simulink model "PMSM_SMC2"  (R2022b)
settings: Solver=ode23tb  StartTime=0.0  StopTime=1  FixedStep=Ts  RelTol=1e-4  EnableMultiTasking=on
InitFcn:
  | Ts = 10e-6;
  | 
  | R = 2.875;
  | Ld = 8.2e-3;
  | Lq = 8.2e-3;
  | Pn = 4;
  | flux = 0.175;
  | alpha1=15;
  | alpha2=9;
  | e=0.0005;
  | B = 0;
  | J = 0.003;
  | a=-(B/J);
  | b=(3*Pn*flux)/(2*J);
  | kq1=100;
  | kq2=80;
undefined symbols (not defined in the file): DiscIntNeverNeededParam, k1, k2
libraries: slpidlib x2, simulink x2, spsPermanentMagnetSynchronousMachineLib x1, powerlib_extras x1, spsUniversalBridgeLib x1, spsDCVoltageSourceLib x1, sps_lib x1
(part 1 of 2)
settings Model: Creator=SUN  LastModifiedBy=hl
settings SolverCC: ZeroCrossControl=DisableAll  AlgebraicLoopSolver=TrustRegion
settings DataIOCC: LimitDataPoints=on  SaveFormat=Array  SignalLoggingSaveFormat=ModelDataLogs  ReturnWorkspaceOutputs=off
settings OptimizationCC: ExpressionDepthLimit=2147483647  InitFltsAndDblsToZero=on  LifeSpan=inf
settings DebuggingCC: UnderspecifiedInitializationDetection=Classic  MergeDetectMultiDrivingBlocksExec=none  SolverPrmCheckMsg=warning  FcnCallInpInsideContextMsg=warning  UnconnectedInputMsg=warning  UnconnectedOutputMsg=warning  UnconnectedLineMsg=warning  StateNameClashWarn=warning  SFUnexpectedBacktrackingDiag=warning  SFNoUnconditionalDefaultTransitionDiag=warning  SFMachineParentedDataDiag=warning  ArithmeticOperatorsInVariantConditions=warning
settings HardwareCC: ProdBitPerPointer=32  ProdBitPerSizeT=32  ProdBitPerPtrDiffT=32  ProdLargestAtomicFloat=None  ProdIntDivRoundTo=Undefined  ProdEndianess=Unspecified  ProdWordSize=32  ProdHWDeviceType=32-bit Generic
settings ModelReferenceCC: EnableRefExpFcnMdlSchedulingChecks=on  PropagateSignalLabelsOutOfModel=off
settings SFSimCC: SimUseLocalCustomCode=off  CustomCodeUndefinedFunction=UseInterfaceOnly
settings RTWCC: RTWUseLocalCustomCode=off
settings CodeAppCC: StateflowObjectComments=on
settings GRTTargetCC: TargetLangStandard=C89/C90 (ANSI)  CombineOutputUpdateFcns=off  GRTInterface=on
settings ConfigComp: CovMetricSettings=dw  CovSaveCumulativeToWorkspaceVar=on  CovSaveSingleToWorkspaceVar=on  CovExternalEMLEnable=off  CovSFcnEnable=off
settings SimscapeCC: SimscapeNormalizeSystem=off

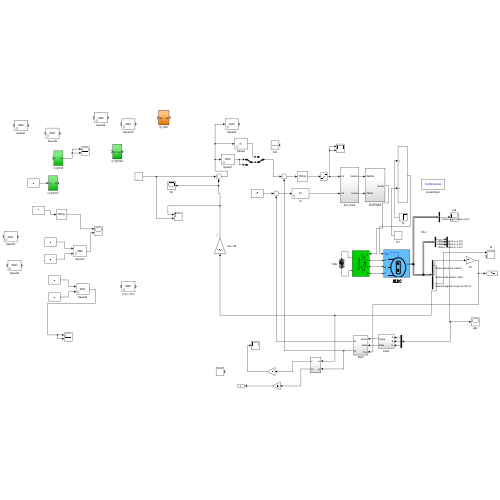
[thumbnail: Simulink's stored preview of the top-level diagram]
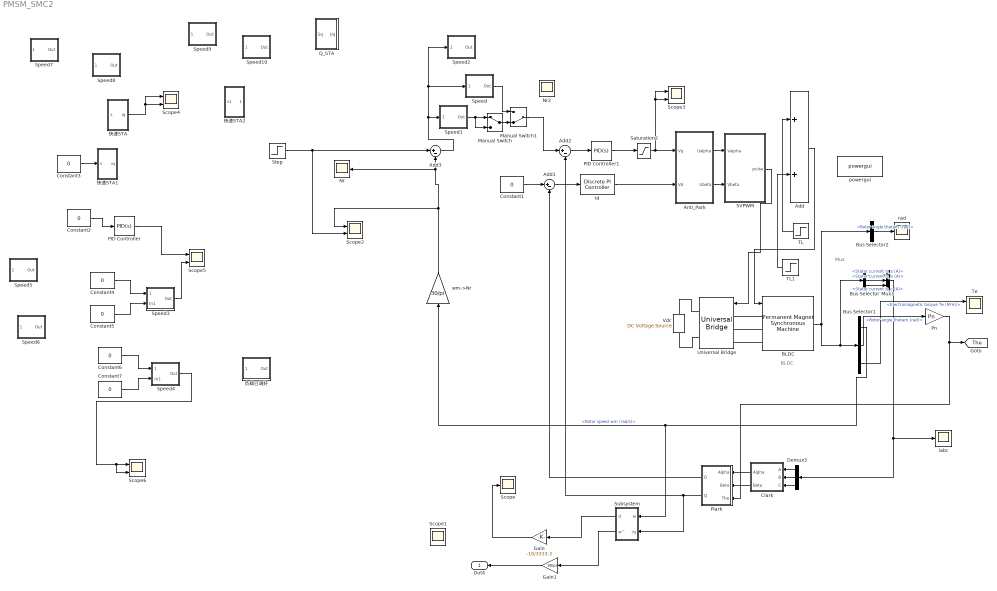
== system PMSM_SMC2 ==
  note: BLDC
  note: Mux
  Add : Sum
  Add1 : Sum  Inputs=|+-
  Add2 : Sum  Inputs=|+-
  Add3 : Sum  Inputs=|+-
  Anti_Park : Subsystem
  BLDC : spsPermanentMagnetSynchronousMachineLib/Permanent Magnet Synchronous Machine  NbPhases=3  FluxDistribution=Sinusoidal  RotorType=Salient-pole  MechanicalLoad=Torque Tm  PresetModel=No  ShowDetailedParameters=on  MeasurementBus=off  Resistance=2.875  Inductance=8.5e-3  dqInductances=[8.5e-3,8.5e-3]  La=0.000835  MachineConstant=Flux linkage established by magnets (V.s)  Flux=0.175  VoltageCst=126.966  TorqueCst=1.05  Flat=120  Mechanical=[0.003 0.008 4 0]  PolePairs=3  InitialConditions=[0,0, 0,0]  InitialConditions5ph=[0 0 0 0 0 0]  RefAngle=Aligned with phase A axis (original Park)  IterativeDiscreteModel=Trapezoidal non iterative  TsBlock=-1  TsPowergui=0
  Bus Selector : BusSelector  OutputSignals=Stator current is_a (A),Stator current is_b (A),Stator current is_c (A)
  Bus Selector1 : BusSelector  OutputSignals=Rotor speed wm (rad/s),Rotor angle thetam (rad),Electromagnetic torque Te (N*m)
  Bus Selector2 : BusSelector  OutputSignals=Rotor angle thetam (rad)
  Clark : Subsystem
  Constant{1..7} (7 alike) : Constant  Value=0
  Demux3 : Demux  Outputs=3
  Gain : Gain  Gain=-10/3333.3
  Gain1 : Gain  Gain=30/pi
  Id : powerlib_extras/Discrete  Control Blocks/Discrete PI Controller  Kp=Ld*2000  Ki=R*2000  Par_Limits=[311*0.9*sqrt(1/3) -311*0.9*sqrt(1/3)]  Init=0  Ts=Ts
  Manual Switch : ManualSwitch
  Manual Switch1 : ManualSwitch  CurrentSetting=0
  Mux3 : Mux  Inputs=3
  Nr : Scope
  Nr2 : Scope
  PID Controller : slpidlib/PID Controller  Controller=PID  Form=Parallel  TimeDomain=Continuous-time  UseExternalTs=off  SampleTime=-1  IntegratorMethod=Forward Euler  FilterMethod=Forward Euler  ControllerParametersSource=internal  P=60  I=10  UseKiTs=off  D=0  N=100  UseFilter=on  TunerSelectOption=Transfer Function Based (PID Tuner App)  InitialConditionSource=internal  InitialConditionForIntegrator=0  InitialConditionForFilter=0  DifferentiatorICPrevScaledInput=0  ExternalReset=none  TrackingMode=off  Kt=1  LimitOutput=off  SatLimitsSource=internal  UpperSaturationLimit=inf  LowerSaturationLimit=-inf  LinearizeAsGain=on  AntiWindupMode=none  Kb=1  LimitIntegrator=off  UpperIntegratorSaturationLimit=inf  LowerIntegratorSaturationLimit=-inf  POutMin=[]  POutMax=[]  IOutMin=[]  IOutMax=[]  DOutMin=[]  DOutMax=[]  NOutMin=[]  NOutMax=[]  SumOutMin=[]  SumOutMax=[]  SaturationOutMin=[]  SaturationOutMax=[]  PParamMin=[]  PParamMax=[]  IParamMin=[]  IParamMax=[]  DParamMin=[]  DParamMax=[]  NParamMin=[]  NParamMax=[]  KbParamMin=[]  KbParamMax=[]  KtParamMin=[]  KtParamMax=[]  KbOutMin=[]  KbOutMax=[]  KtOutMin=[]  KtOutMax=[]  IntegratorOutMin=[]  IntegratorOutMax=[]  FilterOutMin=[]  FilterOutMax=[]  SumI1OutMin=[]  SumI1OutMax=[]  SumI2OutMin=[]  SumI2OutMax=[]  SumI3OutMin=[]  SumI3OutMax=[]  SumI4OutMin=[]  SumI4OutMax=[]  SumDOutMin=[]  SumDOutMax=[]  DifferentiatorOutMin=[]  DifferentiatorOutMax=[]  FilterDiffOutCoefMin=[]  FilterDiffOutCoefMax=[]  ReciprocalOutMin=[]  ReciprocalOutMax=[]  SumDenOutMin=[]  SumDenOutMax=[]  SumNumOutMin=[]  SumNumOutMax=[]  DivideOutMin=[]  DivideOutMax=[]  UdiffTsProdOutMin=[]  UdiffTsProdOutMax=[]  NTsProdOutMin=[]  NTsProdOutMax=[]  UintegralTsProdOutMin=[]  UintegralTsProdOutMax=[]  UngainTsProdOutMin=[]  UngainTsProdOutMax=[]  ClampingZeroOutDataTypeStr=Inherit: Inherit via back propagation  ClampingZeroOutMin=[]  ClampingZeroOutMax=[]  FilterDenConstantOutDataTypeStr=Inherit: Inherit via back propagation  FilterDenConstantOutMin=[]  FilterDenConstantOutMax=[]  PCopyOutDataTypeStr=Inherit: Inherit via back propagation  PCopyOutMin=[]  PCopyOutMax=[]  NCopyOutDataTypeStr=Inherit: Inherit via back propagation  NCopyOutMin=[]  NCopyOutMax=[]  IntegratorContinuousStateAttributes=''  IntegratorStateMustResolveToSignalObject=off  IntegratorRTWStateStorageClass=Auto  FilterContinuousStateAttributes=''  FilterStateMustResolveToSignalObject=off  FilterRTWStateStorageClass=Auto  ParallelPVariant=InternalParameters  IdealPVariant=Disabled  IVariant=InternalParameters  DVariant=InternalParameters  IntegratorVariant=Continuous  SatVariant=Disabled  AWVariant=Passthrough  PCopyVariant=Disabled  TRVariant=Disabled  FdbkBlocksVariant=Forward  IdealPFdbkVariant=Disabled  SatFdbkVariant=Disabled  DerivativeFilterVariant=ContFilter  NVariant=InternalParameters  NCopyVariant=Disabled  FilterICVariant=InternalICsFilter  IntegratorICVariant=InternalICs  ExternalResetVariant=Disabled  TRSumVariant=Passthrough  SumFdbkVariant=Disabled  SumVariant=Sum_PID  TsampFilterVariant=InternalTs  TsampNgainVariant=Passthrough  TsampIntegralVariant=Passthrough  ExternalSaturationOutDataTypeStr=Inherit: Same as second input
  PID Controller1 : slpidlib/PID Controller  Controller=PID  Form=Parallel  TimeDomain=Continuous-time  UseExternalTs=off  SampleTime=-1  IntegratorMethod=Forward Euler  FilterMethod=Forward Euler  ControllerParametersSource=internal  P=60  I=10  UseKiTs=off  D=0  N=100  UseFilter=on  TunerSelectOption=Transfer Function Based (PID Tuner App)  InitialConditionSource=internal  InitialConditionForIntegrator=0  InitialConditionForFilter=0  DifferentiatorICPrevScaledInput=0  ExternalReset=none  TrackingMode=off  Kt=1  LimitOutput=off  SatLimitsSource=internal  UpperSaturationLimit=inf  LowerSaturationLimit=-inf  LinearizeAsGain=on  AntiWindupMode=none  Kb=1  LimitIntegrator=off  UpperIntegratorSaturationLimit=inf  LowerIntegratorSaturationLimit=-inf  POutMin=[]  POutMax=[]  IOutMin=[]  IOutMax=[]  DOutMin=[]  DOutMax=[]  NOutMin=[]  NOutMax=[]  SumOutMin=[]  SumOutMax=[]  SaturationOutMin=[]  SaturationOutMax=[]  PParamMin=[]  PParamMax=[]  IParamMin=[]  IParamMax=[]  DParamMin=[]  DParamMax=[]  NParamMin=[]  NParamMax=[]  KbParamMin=[]  KbParamMax=[]  KtParamMin=[]  KtParamMax=[]  KbOutMin=[]  KbOutMax=[]  KtOutMin=[]  KtOutMax=[]  IntegratorOutMin=[]  IntegratorOutMax=[]  FilterOutMin=[]  FilterOutMax=[]  SumI1OutMin=[]  SumI1OutMax=[]  SumI2OutMin=[]  SumI2OutMax=[]  SumI3OutMin=[]  SumI3OutMax=[]  SumI4OutMin=[]  SumI4OutMax=[]  SumDOutMin=[]  SumDOutMax=[]  DifferentiatorOutMin=[]  DifferentiatorOutMax=[]  FilterDiffOutCoefMin=[]  FilterDiffOutCoefMax=[]  ReciprocalOutMin=[]  ReciprocalOutMax=[]  SumDenOutMin=[]  SumDenOutMax=[]  SumNumOutMin=[]  SumNumOutMax=[]  DivideOutMin=[]  DivideOutMax=[]  UdiffTsProdOutMin=[]  UdiffTsProdOutMax=[]  NTsProdOutMin=[]  NTsProdOutMax=[]  UintegralTsProdOutMin=[]  UintegralTsProdOutMax=[]  UngainTsProdOutMin=[]  UngainTsProdOutMax=[]  ClampingZeroOutDataTypeStr=Inherit: Inherit via back propagation  ClampingZeroOutMin=[]  ClampingZeroOutMax=[]  FilterDenConstantOutDataTypeStr=Inherit: Inherit via back propagation  FilterDenConstantOutMin=[]  FilterDenConstantOutMax=[]  PCopyOutDataTypeStr=Inherit: Inherit via back propagation  PCopyOutMin=[]  PCopyOutMax=[]  NCopyOutDataTypeStr=Inherit: Inherit via back propagation  NCopyOutMin=[]  NCopyOutMax=[]  IntegratorContinuousStateAttributes=''  IntegratorStateMustResolveToSignalObject=off  IntegratorRTWStateStorageClass=Auto  FilterContinuousStateAttributes=''  FilterStateMustResolveToSignalObject=off  FilterRTWStateStorageClass=Auto  ParallelPVariant=InternalParameters  IdealPVariant=Disabled  IVariant=InternalParameters  DVariant=InternalParameters  IntegratorVariant=Continuous  SatVariant=Disabled  AWVariant=Passthrough  PCopyVariant=Disabled  TRVariant=Disabled  FdbkBlocksVariant=Forward  IdealPFdbkVariant=Disabled  SatFdbkVariant=Disabled  DerivativeFilterVariant=ContFilter  NVariant=InternalParameters  NCopyVariant=Disabled  FilterICVariant=InternalICsFilter  IntegratorICVariant=InternalICs  ExternalResetVariant=Disabled  TRSumVariant=Passthrough  SumFdbkVariant=Disabled  SumVariant=Sum_PID  TsampFilterVariant=InternalTs  TsampNgainVariant=Passthrough  TsampIntegralVariant=Passthrough  ExternalSaturationOutDataTypeStr=Inherit: Same as second input
  Plark : Subsystem
  Pn : Gain  Gain=Pn
  Q_STA : Subsystem
  SVPWM : Subsystem
  Saturation2 : Saturate  UpperLimit=380  LowerLimit=-400  SampleTime=Ts
  Scope : Scope
  Scope1 : Scope
  Scope{2..6} (5 alike) : Scope  NumInputPorts=2
  Speed : Subsystem  AncestorBlock=|  DialogController=POWERSYS.PowerSysDialog  mask(Discrete PI Controller){Kpw=0.14, Kiw=0.14*50, Ba=0.013, Par_Limits=[30 -30], Init=0, Ts=Ts}
      | powerlib_extras/Discrete 
      | Control Blocks/Discrete
      | PI Controller
      mask prompts: Kpw "Proportional gain (Kp):"; Kiw "Integral gain (Ki):"; Ba "feedback gain (Ba)"; Par_Limits "Output limits: [ Upper   Lower ]"; Init "Output initial value:"; Ts "Sample time:"
      mask help: This block implements a discrete PI controller.
      mask init:
      | UpperLimit=Par_Limits(1);
      | LowerLimit=Par_Limits(2);
      | power_initmask();
      settings: LibrarySourceBlock=|
      | powerlib_extras/Discrete
      | Control Blocks/Discrete
      | PI Controller
      mask Help: This block is part of a subset of blocks in the Extras library that does not have documentation associated with it, other than the block mask description.
      mask Display: disp('PI');
  Speed1 : Subsystem  AncestorBlock=|  DialogController=POWERSYS.PowerSysDialog  mask(Discrete PI Controller){C=294.3, Mu=200, q=500, Par_Limits=[30 -30], Init=0, Ts=Ts}
      | powerlib_extras/Discrete 
      | Control Blocks/Discrete
      | PI Controller
      mask prompts: C "Gain (c):"; Mu "Gain (Mu):"; q "Gain (q)"; Par_Limits "Output limits: [ Upper   Lower ]"; Init "Output initial value:"; Ts "Sample time:"
      mask help: This block implements a discrete PI controller.
      mask init:
      | UpperLimit=Par_Limits(1);
      | LowerLimit=Par_Limits(2);
      | power_initmask();
      settings: LibrarySourceBlock=|
      | powerlib_extras/Discrete
      | Control Blocks/Discrete
      | PI Controller
      mask Help: This block is part of a subset of blocks in the Extras library that does not have documentation associated with it, other than the block mask description.
      mask Display: disp('SMC');
  Speed10 : Subsystem  AncestorBlock=|  DialogController=POWERSYS.PowerSysDialog  mask(Discrete PI Controller){C=294.3, Mu=200, q=500, Par_Limits=[30 -30], Init=0, Ts=Ts}
      | powerlib_extras/Discrete 
      | Control Blocks/Discrete
      | PI Controller
      mask prompts: C "Gain (c):"; Mu "Gain (Mu):"; q "Gain (q)"; Par_Limits "Output limits: [ Upper   Lower ]"; Init "Output initial value:"; Ts "Sample time:"
      mask help: This block implements a discrete PI controller.
      mask init:
      | UpperLimit=Par_Limits(1);
      | LowerLimit=Par_Limits(2);
      | power_initmask();
      settings: LibrarySourceBlock=|
      | powerlib_extras/Discrete
      | Control Blocks/Discrete
      | PI Controller
      mask Help: This block is part of a subset of blocks in the Extras library that does not have documentation associated with it, other than the block mask description.
      mask Display: disp('SMC');
  Speed2 : Subsystem  AncestorBlock=|  DialogController=POWERSYS.PowerSysDialog  mask(Discrete PI Controller){C=50, Mu=500, q=1000, Par_Limits=[30 -30], Init=0, Ts=Ts}
      | powerlib_extras/Discrete 
      | Control Blocks/Discrete
      | PI Controller
      mask prompts: C "Gain (c):"; Mu "Gain (Mu):"; q "Gain (q)"; Par_Limits "Output limits: [ Upper   Lower ]"; Init "Output initial value:"; Ts "Sample time:"
      mask help: This block implements a discrete PI controller.
      mask init:
      | UpperLimit=Par_Limits(1);
      | LowerLimit=Par_Limits(2);
      | power_initmask();
      settings: LibrarySourceBlock=|
      | powerlib_extras/Discrete
      | Control Blocks/Discrete
      | PI Controller
      mask Help: This block is part of a subset of blocks in the Extras library that does not have documentation associated with it, other than the block mask description.
      mask Display: disp('SMC');
  Speed3 : Subsystem  AncestorBlock=|  DialogController=POWERSYS.PowerSysDialog  mask(Discrete PI Controller){C=605, Mu=200, q=410, Par_Limits=[30 -30], Init=0, Ts=Ts}
      | powerlib_extras/Discrete 
      | Control Blocks/Discrete
      | PI Controller
      mask prompts: C "Gain (c):"; Mu "Gain (Mu):"; q "Gain (q)"; Par_Limits "Output limits: [ Upper   Lower ]"; Init "Output initial value:"; Ts "Sample time:"
      mask help: This block implements a discrete PI controller.
      mask init:
      | UpperLimit=Par_Limits(1);
      | LowerLimit=Par_Limits(2);
      | power_initmask();
      settings: LibrarySourceBlock=|
      | powerlib_extras/Discrete
      | Control Blocks/Discrete
      | PI Controller
      mask Help: This block is part of a subset of blocks in the Extras library that does not have documentation associated with it, other than the block mask description.
      mask Display: disp('SMC');
  Speed4 : Subsystem  AncestorBlock=|  DialogController=POWERSYS.PowerSysDialog  mask(Discrete PI Controller){C=600, Mu=200, q=403.81, Par_Limits=[30 -30], Init=0, Ts=Ts}
      | powerlib_extras/Discrete 
      | Control Blocks/Discrete
      | PI Controller
      mask prompts: C "Gain (c):"; Mu "Gain (Mu):"; q "Gain (q)"; Par_Limits "Output limits: [ Upper   Lower ]"; Init "Output initial value:"; Ts "Sample time:"
      mask help: This block implements a discrete PI controller.
      mask init:
      | UpperLimit=Par_Limits(1);
      | LowerLimit=Par_Limits(2);
      | power_initmask();
      settings: LibrarySourceBlock=|
      | powerlib_extras/Discrete
      | Control Blocks/Discrete
      | PI Controller
      mask Help: This block is part of a subset of blocks in the Extras library that does not have documentation associated with it, other than the block mask description.
      mask Display: disp('SMC');
  Speed5 : Subsystem  AncestorBlock=|  DialogController=POWERSYS.PowerSysDialog  mask(Discrete PI Controller){C=370, Mu=200, q=500, Par_Limits=[30 -30], Init=0, Ts=Ts}
      | powerlib_extras/Discrete 
      | Control Blocks/Discrete
      | PI Controller
      mask prompts: C "Gain (c):"; Mu "Gain (Mu):"; q "Gain (q)"; Par_Limits "Output limits: [ Upper   Lower ]"; Init "Output initial value:"; Ts "Sample time:"
      mask help: This block implements a discrete PI controller.
      mask init:
      | UpperLimit=Par_Limits(1);
      | LowerLimit=Par_Limits(2);
      | power_initmask();
      settings: LibrarySourceBlock=|
      | powerlib_extras/Discrete
      | Control Blocks/Discrete
      | PI Controller
      mask Help: This block is part of a subset of blocks in the Extras library that does not have documentation associated with it, other than the block mask description.
      mask Display: disp('SMC');
  Speed6 : Subsystem  AncestorBlock=|  DialogController=POWERSYS.PowerSysDialog  mask(Discrete PI Controller){C=500, Mu=200, q=300, Par_Limits=[30 -30], Init=0, Ts=Ts}
      | powerlib_extras/Discrete 
      | Control Blocks/Discrete
      | PI Controller
      mask prompts: C "Gain (c):"; Mu "Gain (Mu):"; q "Gain (q)"; Par_Limits "Output limits: [ Upper   Lower ]"; Init "Output initial value:"; Ts "Sample time:"
      mask help: This block implements a discrete PI controller.
      mask init:
      | UpperLimit=Par_Limits(1);
      | LowerLimit=Par_Limits(2);
      | power_initmask();
      settings: LibrarySourceBlock=|
      | powerlib_extras/Discrete
      | Control Blocks/Discrete
      | PI Controller
      mask Help: This block is part of a subset of blocks in the Extras library that does not have documentation associated with it, other than the block mask description.
      mask Display: disp('SMC');
  Speed7 : Subsystem  AncestorBlock=|  DialogController=POWERSYS.PowerSysDialog  mask(Discrete PI Controller){C=195, Mu=200, q=400, Par_Limits=[30 -30], Init=0, Ts=Ts}
      | powerlib_extras/Discrete 
      | Control Blocks/Discrete
      | PI Controller
      mask prompts: C "Gain (c):"; Mu "Gain (Mu):"; q "Gain (q)"; Par_Limits "Output limits: [ Upper   Lower ]"; Init "Output initial value:"; Ts "Sample time:"
      mask help: This block implements a discrete PI controller.
      mask init:
      | UpperLimit=Par_Limits(1);
      | LowerLimit=Par_Limits(2);
      | power_initmask();
      settings: LibrarySourceBlock=|
      | powerlib_extras/Discrete
      | Control Blocks/Discrete
      | PI Controller
      mask Help: This block is part of a subset of blocks in the Extras library that does not have documentation associated with it, other than the block mask description.
      mask Display: disp('SMC');
  Speed8 : Subsystem  AncestorBlock=|  DialogController=POWERSYS.PowerSysDialog  mask(Discrete PI Controller){C=195, Mu=200, q=300, Par_Limits=[30 -30], Init=0, Ts=Ts}
      | powerlib_extras/Discrete 
      | Control Blocks/Discrete
      | PI Controller
      mask prompts: C "Gain (c):"; Mu "Gain (Mu):"; q "Gain (q)"; Par_Limits "Output limits: [ Upper   Lower ]"; Init "Output initial value:"; Ts "Sample time:"
      mask help: This block implements a discrete PI controller.
      mask init:
      | UpperLimit=Par_Limits(1);
      | LowerLimit=Par_Limits(2);
      | power_initmask();
      settings: LibrarySourceBlock=|
      | powerlib_extras/Discrete
      | Control Blocks/Discrete
      | PI Controller
      mask Help: This block is part of a subset of blocks in the Extras library that does not have documentation associated with it, other than the block mask description.
      mask Display: disp('SMC');
  Speed9 : Subsystem  AncestorBlock=|  DialogController=POWERSYS.PowerSysDialog  mask(Discrete PI Controller){C=150, Mu=200, q=200, Par_Limits=[30 -30], Init=0, Ts=Ts}
      | powerlib_extras/Discrete 
      | Control Blocks/Discrete
      | PI Controller
      mask prompts: C "Gain (c):"; Mu "Gain (Mu):"; q "Gain (q)"; Par_Limits "Output limits: [ Upper   Lower ]"; Init "Output initial value:"; Ts "Sample time:"
      mask help: This block implements a discrete PI controller.
      mask init:
      | UpperLimit=Par_Limits(1);
      | LowerLimit=Par_Limits(2);
      | power_initmask();
      settings: LibrarySourceBlock=|
      | powerlib_extras/Discrete
      | Control Blocks/Discrete
      | PI Controller
      mask Help: This block is part of a subset of blocks in the Extras library that does not have documentation associated with it, other than the block mask description.
      mask Display: disp('SMC');
  Step : Step  Time=0.6  Before=500  After=1000  SampleTime=0
  Subsystem : Subsystem
  TL : Step  Time=0.3  After=10  SampleTime=0
  TL1 : Step  Time=0.8  After=-5  SampleTime=0
  Te : Scope  NumInputPorts=2
  Universal Bridge : spsUniversalBridgeLib/Universal Bridge  Arms=3  SnubberResistance=1e5  SnubberCapacitance=inf  Device=IGBT / Diodes  Ron=1e-3  Lon=0  ForwardVoltages="[  0  0  ]"  ForwardVoltage=0  GTOparameters=[ 10e-6 , 20e-6 ]  IGBTparameters=[ 1e-6 , 2e-6 ]  Measurements=None  Measurements_2=None  converterType=Rectifier
  Vdc : spsDCVoltageSourceLib/DC Voltage Source  Amplitude=311  Measurements=None
  iabc : Scope
  powergui : sps_lib/powergui  SimulationMode=Continuous  SampleTime=Ts  frequency=60  Iterations=50  frequencyindice=0  Pbase=100e6  ErrMax=1e-4  UnitsV=kV  UnitsW=MW  buscounter=0  FunctionMessages=off  echomessages=off  EnableUseOfTLC=off  CurrentSourceSwitches=on  DisableSnubberDevices=off  DisableRonSwitches=off  DisableVfSwitches=off  DisplayEquations=off  AutomaticDiscreteSolvers=off  SolverType=Tustin/Backward Euler (TBE)  Interpol=off  ExternalGateDelay=off  methode=off  Ts=0  x0status=blocks  SPID=off  SwTol=0  HookPort=off  NonlinearTolerance=1e-4  nMaxIteration=100  ContinueOnMaxIteration=off  RestoreLinks=warning  ResistiveCurrentMeasurement=off  Frange=[0:2:500]  Ylog=off  Xlog=on  ShowGrid=off  save=off  variable=ZData  structure=0  ZoomFFT=on  StartTime=0.0  cycles=1  DisplayStyle=1  fundamental=60  FreqAxis=off  MaxFrequency=1000  frequencyindicesteady=1  RmsSteady=1  display=off
  rad : Scope
  wm->Nr : Gain  Gain=30/pi
  快速STA : Subsystem
  快速STA1 : Subsystem
  快速STA2 : Subsystem
  负载已调好 : Subsystem  AncestorBlock=|  DialogController=POWERSYS.PowerSysDialog  mask(Discrete PI Controller){C=515, Mu=200, q=450, Par_Limits=[30 -30], Init=0, Ts=Ts}
      | powerlib_extras/Discrete 
      | Control Blocks/Discrete
      | PI Controller
      mask prompts: C "Gain (c):"; Mu "Gain (Mu):"; q "Gain (q)"; Par_Limits "Output limits: [ Upper   Lower ]"; Init "Output initial value:"; Ts "Sample time:"
      mask help: This block implements a discrete PI controller.
      mask init:
      | UpperLimit=Par_Limits(1);
      | LowerLimit=Par_Limits(2);
      | power_initmask();
      settings: LibrarySourceBlock=|
      | powerlib_extras/Discrete
      | Control Blocks/Discrete
      | PI Controller
      mask Help: This block is part of a subset of blocks in the Extras library that does not have documentation associated with it, other than the block mask description.
      mask Display: disp('SMC');
  Out4 : Outport
  tag scope: The=global
  wires:
  Constant1/1 -> Add1/1
  wm->Nr/1 -> Add3/2, Nr/1, Scope2/1
  Id/1 -> Anti_Park/2(Vd)
  Pn/1 -> Plark/3(The), [The]
  SVPWM/1(pulse) -> Universal Bridge/1
  Mux3/1 -> Demux3/1, iabc/1
  Anti_Park/1(Ualpha) -> SVPWM/1(Valpha)
  Anti_Park/2(Ubeta) -> SVPWM/2(Vbeta)
  Bus Selector/1 -> Mux3/1  "<Stator current is_a (A)>"
  Bus Selector/3 -> Mux3/3  "<Stator current is_c (A)>"
  Bus Selector/2 -> Mux3/2  "<Stator current is_b (A)>"
  BLDC/1 -> Bus Selector/1, Bus Selector1/1, Bus Selector2/1
  Bus Selector1/3 -> Te/1  "<Electromagnetic torque Te (N*m)>"
  Bus Selector1/2 -> Pn/1  "<Rotor angle thetam (rad)>"
  Bus Selector1/1 -> Subsystem/1(w), wm->Nr/1  "<Rotor speed wm (rad/s)>"
  Bus Selector2/1 -> rad/1  "<Rotor angle thetam (rad)>"
  Add1/1 -> Id/1
  Saturation2/1 -> Anti_Park/1(Vq), Scope3/2, Scope3/1
  TL/1 -> Add/1
  TL1/1 -> Add/2
  Add/1 -> BLDC/1
  Constant2/1 -> PID Controller/1
  PID Controller/1 -> Scope5/1
  快速STA/1(iq) -> Scope4/1, Scope4/2
  Constant4/1 -> Speed3/1(Error)
  Constant5/1 -> Speed3/2(In1)
  Speed3/1(Out) -> Scope5/2
  Step/1 -> Scope2/2, Add3/1
  Constant6/1 -> Speed4/1(Error)
  Constant7/1 -> Speed4/2(In1)
  Speed4/1(Out) -> Scope6/2, Scope6/1
  Constant3/1 -> 快速STA1/1(s)
  Manual Switch/1 -> Manual Switch1/2
  Speed1/1(Out) -> Manual Switch/2, Manual Switch/1
  Demux3/2 -> Clark/2(B)
  Plark/2(Q) -> Add2/2, Subsystem/2(iq)
  Demux3/3 -> Clark/3(C)
  Clark/2(Beta) -> Plark/2(Beta)
  Subsystem/2(w^) -> Gain1/1
  Clark/1(Alpha) -> Plark/1(Alpha)
  Gain1/1 -> Out4/1
  Subsystem/1(d) -> Gain/1
  Demux3/1 -> Clark/1(A)
  Plark/1(D) -> Add1/2
  Gain/1 -> Scope/1
  Manual Switch1/1 -> Add2/1
  Add3/1 -> Speed/1(Error), Speed2/1(Error), Speed1/1(Error)
  Add2/1 -> PID Controller1/1
  PID Controller1/1 -> Saturation2/1
  Speed/1(Out) -> Manual Switch1/1
  connections:
  Universal Bridge/RConn1 -- Vdc/RConn1
  BLDC/LConn3 -- Universal Bridge/LConn3
  BLDC/LConn2 -- Universal Bridge/LConn2
  Universal Bridge/RConn2 -- Vdc/LConn1
  BLDC/LConn1 -- Universal Bridge/LConn1

== system PMSM_SMC2/Anti_Park ==
  Vq : Inport
  Vd : Inport  Port=2
  Fcn : Fcn  Expr=cos(u[1])*u[2]-sin(u[1])*u[3]
  Fcn1 : Fcn  Expr=sin(u[1])*u[2]+cos(u[1])*u[3]
  Mux1 : Mux  Inputs=3
  Ualpha : Outport  VectorParamsAs1DForOutWhenUnconnected=off
  Ubeta : Outport  Port=2  VectorParamsAs1DForOutWhenUnconnected=off
  wires:
  Fcn1/1 -> Ubeta/1
  Fcn/1 -> Ualpha/1
  Mux1/1 -> Fcn/1, Fcn1/1
  Vd/1 -> Mux1/2
  Vq/1 -> Mux1/3
  [The] -> Mux1/1

== system PMSM_SMC2/Clark ==
  A : Inport
  B : Inport  Port=2
  C : Inport  Port=3
  Mux : Mux  Inputs=3
  alpha : Fcn  Expr=(u(1)-0.5*(u(2)+u(3)))*2/3
  beta : Fcn  Expr=sqrt(3)/2*(u(2)-u(3))*2/3
  Alpha : Outport  VectorParamsAs1DForOutWhenUnconnected=off
  Beta : Outport  Port=2  VectorParamsAs1DForOutWhenUnconnected=off
  wires:
  alpha/1 -> Alpha/1
  B/1 -> Mux/2
  C/1 -> Mux/3
  A/1 -> Mux/1
  Mux/1 -> beta/1, alpha/1
  beta/1 -> Beta/1

== system PMSM_SMC2/Plark ==
  Alpha : Inport
  Beta : Inport  Port=2
  The : Inport  Port=3
  Mux : Mux  Inputs=3
  d : Fcn  Expr=u(1)*cos(u(3))+u(2)*sin(u(3))
  q : Fcn  Expr=-u(1)*sin(u(3))+u(2)*cos(u(3))
  D : Outport  VectorParamsAs1DForOutWhenUnconnected=off
  Q : Outport  Port=2  VectorParamsAs1DForOutWhenUnconnected=off
  wires:
  d/1 -> D/1
  Beta/1 -> Mux/2
  The/1 -> Mux/3
  Alpha/1 -> Mux/1
  Mux/1 -> q/1, d/1
  q/1 -> Q/1

== system PMSM_SMC2/Q_STA ==
  Sq : Inport
  Abs : Abs  SaturateOnIntegerOverflow=off
  Add : Sum
  Constant : Constant  Value=0.5
  Discrete-Time Integrator : DiscreteIntegrator  ICPrevOutput=DiscIntNeverNeededParam  ICPrevScaledInput=DiscIntNeverNeededParam
  Gain : Gain  Gain=100
  Gain1 : Gain  Gain=300
  Math Function : Math  Operator=pow  SignedPower=on
  Product : Product
  Sign : Signum
  Uq : Outport
  wires:
  Add/1 -> Uq/1
  Gain1/1 -> Discrete-Time Integrator/1
  Discrete-Time Integrator/1 -> Add/2
  Gain/1 -> Add/1
  Sq/1 -> Sign/1, Abs/1
  Product/1 -> Gain/1
  Sign/1 -> Gain1/1, Product/2
  Constant/1 -> Math Function/2
  Math Function/1 -> Product/1
  Abs/1 -> Math Function/1

== system PMSM_SMC2/SVPWM ==
  Valpha : Inport
  Vbeta : Inport  Port=2
  PWM : Subsystem
  Repeating Sequence : simulink/Sources/Repeating Sequence  rep_seq_t=[0 0.00005 0.0001]  rep_seq_y=[0 0.00005 0]
  Sector Caculate : Subsystem
  T1T1 Caculate : Subsystem
  Tcm Caculate : Subsystem
  Tpwm : Constant  Value=0.0001
  Vdc : Constant  Value=311
  XYZ Caculate : Subsystem
  pulse : Outport  VectorParamsAs1DForOutWhenUnconnected=off
  wires:
  PWM/1(PWM) -> pulse/1
  Repeating Sequence/1 -> PWM/1(In)
  Vbeta/1 -> XYZ Caculate/2(Ubeta), Sector Caculate/2(Ubeta)
  T1T1 Caculate/1(T1) -> Tcm Caculate/2(T1)
  Valpha/1 -> XYZ Caculate/1(Ualpha), Sector Caculate/1(Ualpha)
  T1T1 Caculate/2(T2) -> Tcm Caculate/3(T2)
  Sector Caculate/1("N ") -> Tcm Caculate/1(N), T1T1 Caculate/1(N)
  XYZ Caculate/1(XYZ) -> T1T1 Caculate/2(XYZ)
  Tpwm/1 -> XYZ Caculate/3(Ts), Tcm Caculate/4(Tpwm), T1T1 Caculate/3(Tpwm)
  Vdc/1 -> XYZ Caculate/4(Udc)
  Tcm Caculate/1(Tcm1 Tcm2 Tcm3) -> PWM/2(Tcm123)

== system PMSM_SMC2/Speed ==
  note: Discrete PID Controller
  note: Pierre Giroux, Gilbert Sybille
      | Power System Simulation Laboratory
      | IREQ, Hydro-Quebc
  Error : Inport  SampleTime=Ts
  Discrete-Time Integrator : DiscreteIntegrator  InitialCondition=Init  SampleTime=Ts  LimitOutput=on  UpperSaturationLimit=UpperLimit  LowerSaturationLimit=LowerLimit  ICPrevOutput=DiscIntNeverNeededParam  ICPrevScaledInput=DiscIntNeverNeededParam
  Kp1 : Gain  Gain=Ba  SaturateOnIntegerOverflow=on  SampleTime=Ts  OutDataTypeStr=Inherit: Same as input  ParamDataTypeStr=Inherit: Same as input
  Kp4 : Gain  Gain=Kpw  SaturateOnIntegerOverflow=on  SampleTime=Ts  OutDataTypeStr=Inherit: Same as input  ParamDataTypeStr=Inherit: Same as input
  Kp5 : Gain  Gain=Kiw  SaturateOnIntegerOverflow=on  SampleTime=Ts  OutDataTypeStr=Inherit: Same as input  ParamDataTypeStr=Inherit: Same as input
  Saturation2 : Saturate  UpperLimit=UpperLimit  LowerLimit=LowerLimit  SampleTime=Ts
  Sum6 : Sum  Inputs=++-  InputSameDT=on  SaturateOnIntegerOverflow=on  SampleTime=Ts  OutDataTypeStr=Inherit: Same as first input
  Zero-Order Hold : ZeroOrderHold  SampleTime=Ts
  Out : Outport  SampleTime=Ts  InitialOutput=0  VectorParamsAs1DForOutWhenUnconnected=off
  wires:
  Error/1 -> Kp1/1, Kp5/1, Kp4/1
  Zero-Order Hold/1 -> Sum6/1
  Saturation2/1 -> Out/1
  Discrete-Time Integrator/1 -> Sum6/2
  Kp4/1 -> Zero-Order Hold/1
  Kp5/1 -> Discrete-Time Integrator/1
  Sum6/1 -> Saturation2/1
  Kp1/1 -> Sum6/3

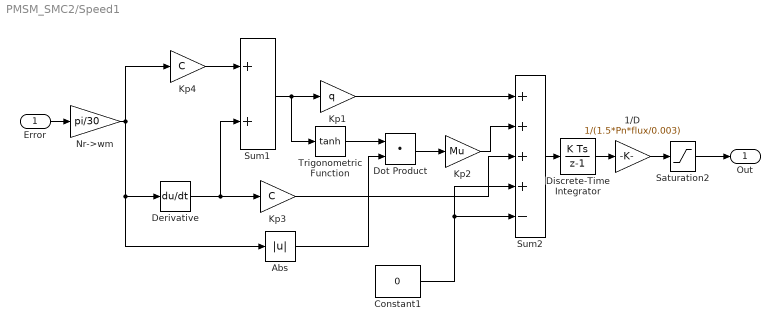
== system PMSM_SMC2/Speed1 ==
  Error : Inport  SampleTime=Ts
  1/D : Gain  Gain=1/(1.5*Pn*flux/0.003)  SaturateOnIntegerOverflow=on  SampleTime=Ts  OutDataTypeStr=Inherit: Same as input  ParamDataTypeStr=Inherit: Same as input
  Abs : Abs  SaturateOnIntegerOverflow=off
  Constant1 : Constant  Value=0
  Derivative : Derivative
  Discrete-Time Integrator : DiscreteIntegrator  InitialCondition=0.001  SampleTime=Ts  ICPrevOutput=DiscIntNeverNeededParam  ICPrevScaledInput=DiscIntNeverNeededParam
  Dot Product : DotProduct  OutDataTypeStr=Inherit: Inherit via internal rule
  Kp1 : Gain  Gain=q  SaturateOnIntegerOverflow=on  SampleTime=Ts  OutDataTypeStr=Inherit: Same as input  ParamDataTypeStr=Inherit: Same as input
  Kp2 : Gain  Gain=Mu  SaturateOnIntegerOverflow=on  SampleTime=Ts  OutDataTypeStr=Inherit: Same as input  ParamDataTypeStr=Inherit: Same as input
  Kp3 : Gain  Gain=C  SaturateOnIntegerOverflow=on  SampleTime=Ts  OutDataTypeStr=Inherit: Same as input  ParamDataTypeStr=Inherit: Same as input
  Kp4 : Gain  Gain=C  SaturateOnIntegerOverflow=on  SampleTime=Ts  OutDataTypeStr=Inherit: Same as input  ParamDataTypeStr=Inherit: Same as input
  Nr->wm : Gain  Gain=pi/30  SaturateOnIntegerOverflow=on  SampleTime=Ts  OutDataTypeStr=Inherit: Same as input  ParamDataTypeStr=Inherit: Same as input
  Saturation2 : Saturate  UpperLimit=UpperLimit  LowerLimit=LowerLimit  SampleTime=Ts
  Sum1 : Sum  InputSameDT=on  SaturateOnIntegerOverflow=on  SampleTime=Ts  OutDataTypeStr=Inherit: Same as first input
  Sum2 : Sum  Inputs=++++-  InputSameDT=on  SaturateOnIntegerOverflow=on  SampleTime=Ts  OutDataTypeStr=Inherit: Same as first input
  Trigonometric Function : Trigonometry  Operator=tanh
  Out : Outport  SampleTime=Ts  InitialOutput=0  VectorParamsAs1DForOutWhenUnconnected=off
  wires:
  Kp4/1 -> Sum1/1
  Saturation2/1 -> Out/1
  Error/1 -> Nr->wm/1
  Kp1/1 -> Sum2/1
  Sum1/1 -> Trigonometric Function/1, Kp1/1
  Kp2/1 -> Sum2/2
  Kp3/1 -> Sum2/3
  Nr->wm/1 -> Kp4/1, Abs/1, Derivative/1
  Derivative/1 -> Sum1/2, Kp3/1
  Sum2/1 -> Discrete-Time Integrator/1
  1/D/1 -> Saturation2/1
  Discrete-Time Integrator/1 -> 1/D/1
  Dot Product/1 -> Kp2/1
  Abs/1 -> Dot Product/2
  Trigonometric Function/1 -> Dot Product/1
  Constant1/1 -> Sum2/5, Sum2/4

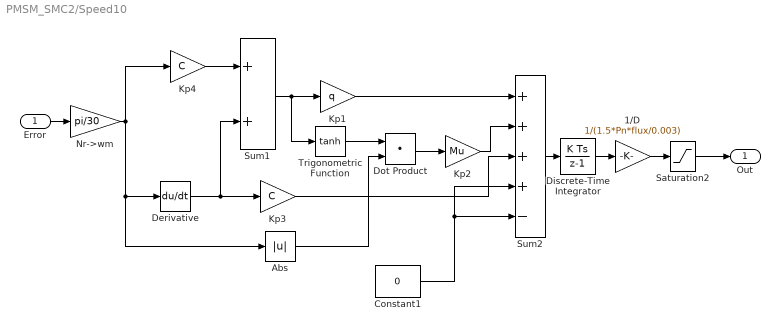
== system PMSM_SMC2/Speed10 ==
  Error : Inport  SampleTime=Ts
  1/D : Gain  Gain=1/(1.5*Pn*flux/0.003)  SaturateOnIntegerOverflow=on  SampleTime=Ts  OutDataTypeStr=Inherit: Same as input  ParamDataTypeStr=Inherit: Same as input
  Abs : Abs  SaturateOnIntegerOverflow=off
  Constant1 : Constant  Value=0
  Derivative : Derivative
  Discrete-Time Integrator : DiscreteIntegrator  InitialCondition=0.001  SampleTime=Ts  ICPrevOutput=DiscIntNeverNeededParam  ICPrevScaledInput=DiscIntNeverNeededParam
  Dot Product : DotProduct  OutDataTypeStr=Inherit: Inherit via internal rule
  Kp1 : Gain  Gain=q  SaturateOnIntegerOverflow=on  SampleTime=Ts  OutDataTypeStr=Inherit: Same as input  ParamDataTypeStr=Inherit: Same as input
  Kp2 : Gain  Gain=Mu  SaturateOnIntegerOverflow=on  SampleTime=Ts  OutDataTypeStr=Inherit: Same as input  ParamDataTypeStr=Inherit: Same as input
  Kp3 : Gain  Gain=C  SaturateOnIntegerOverflow=on  SampleTime=Ts  OutDataTypeStr=Inherit: Same as input  ParamDataTypeStr=Inherit: Same as input
  Kp4 : Gain  Gain=C  SaturateOnIntegerOverflow=on  SampleTime=Ts  OutDataTypeStr=Inherit: Same as input  ParamDataTypeStr=Inherit: Same as input
  Nr->wm : Gain  Gain=pi/30  SaturateOnIntegerOverflow=on  SampleTime=Ts  OutDataTypeStr=Inherit: Same as input  ParamDataTypeStr=Inherit: Same as input
  Saturation2 : Saturate  UpperLimit=UpperLimit  LowerLimit=LowerLimit  SampleTime=Ts
  Sum1 : Sum  InputSameDT=on  SaturateOnIntegerOverflow=on  SampleTime=Ts  OutDataTypeStr=Inherit: Same as first input
  Sum2 : Sum  Inputs=++++-  InputSameDT=on  SaturateOnIntegerOverflow=on  SampleTime=Ts  OutDataTypeStr=Inherit: Same as first input
  Trigonometric Function : Trigonometry  Operator=tanh
  Out : Outport  SampleTime=Ts  InitialOutput=0  VectorParamsAs1DForOutWhenUnconnected=off
  wires:
  Kp4/1 -> Sum1/1
  Saturation2/1 -> Out/1
  Error/1 -> Nr->wm/1
  Kp1/1 -> Sum2/1
  Sum1/1 -> Trigonometric Function/1, Kp1/1
  Kp2/1 -> Sum2/2
  Kp3/1 -> Sum2/3
  Nr->wm/1 -> Kp4/1, Abs/1, Derivative/1
  Derivative/1 -> Sum1/2, Kp3/1
  Sum2/1 -> Discrete-Time Integrator/1
  1/D/1 -> Saturation2/1
  Discrete-Time Integrator/1 -> 1/D/1
  Dot Product/1 -> Kp2/1
  Abs/1 -> Dot Product/2
  Trigonometric Function/1 -> Dot Product/1
  Constant1/1 -> Sum2/5, Sum2/4

== system PMSM_SMC2/Speed2 ==
  Error : Inport  SampleTime=Ts
  1/D : Gain  Gain=1/(1.5*Pn*flux/0.003)  SaturateOnIntegerOverflow=on  SampleTime=Ts  OutDataTypeStr=Inherit: Same as input  ParamDataTypeStr=Inherit: Same as input
  Discrete Derivative : simulink/Discrete/Discrete Derivative  gainval=1.0  ICPrevScaledInput=0.0  OutMin=[]  OutMax=[]  OutDataType=fixdt(1, 16)  OutScaling=2^-10  DoSatur=off
  Discrete-Time Integrator : DiscreteIntegrator  InitialCondition=0.001  SampleTime=Ts  ICPrevOutput=DiscIntNeverNeededParam  ICPrevScaledInput=DiscIntNeverNeededParam
  Kp1 : Gain  Gain=q  SaturateOnIntegerOverflow=on  SampleTime=Ts  OutDataTypeStr=Inherit: Same as input  ParamDataTypeStr=Inherit: Same as input
  Kp2 : Gain  Gain=Mu  SaturateOnIntegerOverflow=on  SampleTime=Ts  OutDataTypeStr=Inherit: Same as input  ParamDataTypeStr=Inherit: Same as input
  Kp3 : Gain  Gain=C  SaturateOnIntegerOverflow=on  SampleTime=Ts  OutDataTypeStr=Inherit: Same as input  ParamDataTypeStr=Inherit: Same as input
  Kp4 : Gain  Gain=C  SaturateOnIntegerOverflow=on  SampleTime=Ts  OutDataTypeStr=Inherit: Same as input  ParamDataTypeStr=Inherit: Same as input
  Nr->wm : Gain  Gain=pi/30  SaturateOnIntegerOverflow=on  SampleTime=Ts  OutDataTypeStr=Inherit: Same as input  ParamDataTypeStr=Inherit: Same as input
  Saturation2 : Saturate  UpperLimit=UpperLimit  LowerLimit=LowerLimit  SampleTime=Ts
  Sign : Signum
  Sum1 : Sum  InputSameDT=on  SaturateOnIntegerOverflow=on  SampleTime=Ts  OutDataTypeStr=Inherit: Same as first input
  Sum2 : Sum  Inputs=++-  InputSameDT=on  SaturateOnIntegerOverflow=on  SampleTime=Ts  OutDataTypeStr=Inherit: Same as first input
  Out : Outport  SampleTime=Ts  InitialOutput=0
  wires:
  Kp4/1 -> Sum1/1
  Saturation2/1 -> Out/1
  Discrete Derivative/1 -> Kp3/1, Sum1/2
  Sum2/1 -> Discrete-Time Integrator/1
  Error/1 -> Nr->wm/1
  Kp1/1 -> Sum2/1
  Sum1/1 -> Kp1/1, Sign/1
  Kp2/1 -> Sum2/2
  Kp3/1 -> Sum2/3
  1/D/1 -> Saturation2/1
  Discrete-Time Integrator/1 -> 1/D/1
  Nr->wm/1 -> Discrete Derivative/1, Kp4/1
  Sign/1 -> Kp2/1

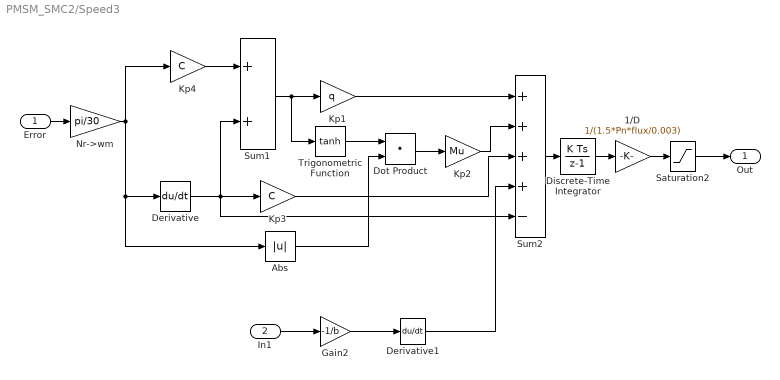
== system PMSM_SMC2/Speed3 ==
  Error : Inport  SampleTime=Ts
  In1 : Inport  Port=2
  1/D : Gain  Gain=1/(1.5*Pn*flux/0.003)  SaturateOnIntegerOverflow=on  SampleTime=Ts  OutDataTypeStr=Inherit: Same as input  ParamDataTypeStr=Inherit: Same as input
  Abs : Abs  SaturateOnIntegerOverflow=off
  Derivative : Derivative
  Derivative1 : Derivative
  Discrete-Time Integrator : DiscreteIntegrator  InitialCondition=0.001  SampleTime=Ts  ICPrevOutput=DiscIntNeverNeededParam  ICPrevScaledInput=DiscIntNeverNeededParam
  Dot Product : DotProduct  OutDataTypeStr=Inherit: Inherit via internal rule
  Gain2 : Gain  Gain=-1/b
  Kp1 : Gain  Gain=q  SaturateOnIntegerOverflow=on  SampleTime=Ts  OutDataTypeStr=Inherit: Same as input  ParamDataTypeStr=Inherit: Same as input
  Kp2 : Gain  Gain=Mu  SaturateOnIntegerOverflow=on  SampleTime=Ts  OutDataTypeStr=Inherit: Same as input  ParamDataTypeStr=Inherit: Same as input
  Kp3 : Gain  Gain=C  SaturateOnIntegerOverflow=on  SampleTime=Ts  OutDataTypeStr=Inherit: Same as input  ParamDataTypeStr=Inherit: Same as input
  Kp4 : Gain  Gain=C  SaturateOnIntegerOverflow=on  SampleTime=Ts  OutDataTypeStr=Inherit: Same as input  ParamDataTypeStr=Inherit: Same as input
  Nr->wm : Gain  Gain=pi/30  SaturateOnIntegerOverflow=on  SampleTime=Ts  OutDataTypeStr=Inherit: Same as input  ParamDataTypeStr=Inherit: Same as input
  Saturation2 : Saturate  UpperLimit=UpperLimit  LowerLimit=LowerLimit  SampleTime=Ts
  Sum1 : Sum  InputSameDT=on  SaturateOnIntegerOverflow=on  SampleTime=Ts  OutDataTypeStr=Inherit: Same as first input
  Sum2 : Sum  Inputs=++++-  InputSameDT=on  SaturateOnIntegerOverflow=on  SampleTime=Ts  OutDataTypeStr=Inherit: Same as first input
  Trigonometric Function : Trigonometry  Operator=tanh
  Out : Outport  SampleTime=Ts  InitialOutput=0  VectorParamsAs1DForOutWhenUnconnected=off
  wires:
  Kp4/1 -> Sum1/1
  Saturation2/1 -> Out/1
  Error/1 -> Nr->wm/1
  Kp1/1 -> Sum2/1
  Sum1/1 -> Trigonometric Function/1, Kp1/1
  Kp2/1 -> Sum2/2
  Kp3/1 -> Sum2/3
  Nr->wm/1 -> Kp4/1, Abs/1, Derivative/1
  Derivative/1 -> Sum2/5, Sum1/2, Kp3/1
  Sum2/1 -> Discrete-Time Integrator/1
  1/D/1 -> Saturation2/1
  Discrete-Time Integrator/1 -> 1/D/1
  Dot Product/1 -> Kp2/1
  Abs/1 -> Dot Product/2
  In1/1 -> Gain2/1
  Gain2/1 -> Derivative1/1
  Derivative1/1 -> Sum2/4
  Trigonometric Function/1 -> Dot Product/1

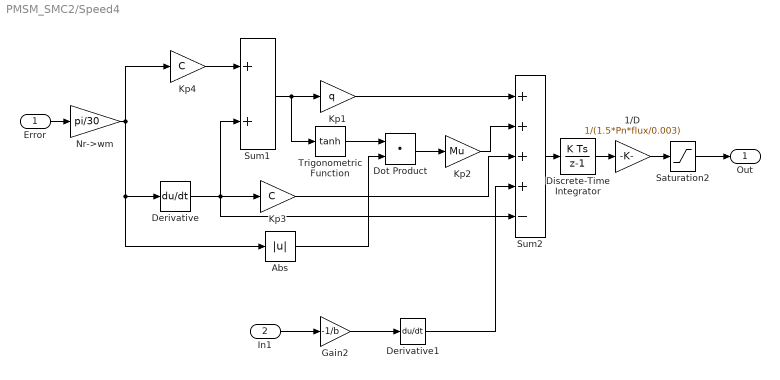
== system PMSM_SMC2/Speed4 ==
  Error : Inport  SampleTime=Ts
  In1 : Inport  Port=2
  1/D : Gain  Gain=1/(1.5*Pn*flux/0.003)  SaturateOnIntegerOverflow=on  SampleTime=Ts  OutDataTypeStr=Inherit: Same as input  ParamDataTypeStr=Inherit: Same as input
  Abs : Abs  SaturateOnIntegerOverflow=off
  Derivative : Derivative
  Derivative1 : Derivative
  Discrete-Time Integrator : DiscreteIntegrator  InitialCondition=0.001  SampleTime=Ts  ICPrevOutput=DiscIntNeverNeededParam  ICPrevScaledInput=DiscIntNeverNeededParam
  Dot Product : DotProduct  OutDataTypeStr=Inherit: Inherit via internal rule
  Gain2 : Gain  Gain=-1/b
  Kp1 : Gain  Gain=q  SaturateOnIntegerOverflow=on  SampleTime=Ts  OutDataTypeStr=Inherit: Same as input  ParamDataTypeStr=Inherit: Same as input
  Kp2 : Gain  Gain=Mu  SaturateOnIntegerOverflow=on  SampleTime=Ts  OutDataTypeStr=Inherit: Same as input  ParamDataTypeStr=Inherit: Same as input
  Kp3 : Gain  Gain=C  SaturateOnIntegerOverflow=on  SampleTime=Ts  OutDataTypeStr=Inherit: Same as input  ParamDataTypeStr=Inherit: Same as input
  Kp4 : Gain  Gain=C  SaturateOnIntegerOverflow=on  SampleTime=Ts  OutDataTypeStr=Inherit: Same as input  ParamDataTypeStr=Inherit: Same as input
  Nr->wm : Gain  Gain=pi/30  SaturateOnIntegerOverflow=on  SampleTime=Ts  OutDataTypeStr=Inherit: Same as input  ParamDataTypeStr=Inherit: Same as input
  Saturation2 : Saturate  UpperLimit=UpperLimit  LowerLimit=LowerLimit  SampleTime=Ts
  Sum1 : Sum  InputSameDT=on  SaturateOnIntegerOverflow=on  SampleTime=Ts  OutDataTypeStr=Inherit: Same as first input
  Sum2 : Sum  Inputs=++++-  InputSameDT=on  SaturateOnIntegerOverflow=on  SampleTime=Ts  OutDataTypeStr=Inherit: Same as first input
  Trigonometric Function : Trigonometry  Operator=tanh
  Out : Outport  SampleTime=Ts  InitialOutput=0  VectorParamsAs1DForOutWhenUnconnected=off
  wires:
  Kp4/1 -> Sum1/1
  Saturation2/1 -> Out/1
  Error/1 -> Nr->wm/1
  Kp1/1 -> Sum2/1
  Sum1/1 -> Trigonometric Function/1, Kp1/1
  Kp2/1 -> Sum2/2
  Kp3/1 -> Sum2/3
  Nr->wm/1 -> Kp4/1, Abs/1, Derivative/1
  Derivative/1 -> Sum2/5, Sum1/2, Kp3/1
  Sum2/1 -> Discrete-Time Integrator/1
  1/D/1 -> Saturation2/1
  Discrete-Time Integrator/1 -> 1/D/1
  Dot Product/1 -> Kp2/1
  Abs/1 -> Dot Product/2
  In1/1 -> Gain2/1
  Gain2/1 -> Derivative1/1
  Derivative1/1 -> Sum2/4
  Trigonometric Function/1 -> Dot Product/1

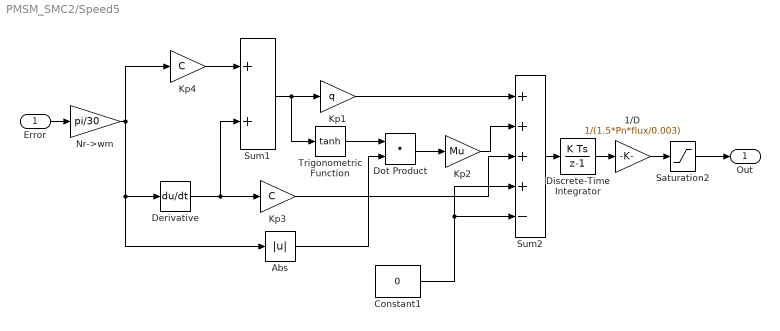
== system PMSM_SMC2/Speed5 ==
  Error : Inport  SampleTime=Ts
  1/D : Gain  Gain=1/(1.5*Pn*flux/0.003)  SaturateOnIntegerOverflow=on  SampleTime=Ts  OutDataTypeStr=Inherit: Same as input  ParamDataTypeStr=Inherit: Same as input
  Abs : Abs  SaturateOnIntegerOverflow=off
  Constant1 : Constant  Value=0
  Derivative : Derivative
  Discrete-Time Integrator : DiscreteIntegrator  InitialCondition=0.001  SampleTime=Ts  ICPrevOutput=DiscIntNeverNeededParam  ICPrevScaledInput=DiscIntNeverNeededParam
  Dot Product : DotProduct  OutDataTypeStr=Inherit: Inherit via internal rule
  Kp1 : Gain  Gain=q  SaturateOnIntegerOverflow=on  SampleTime=Ts  OutDataTypeStr=Inherit: Same as input  ParamDataTypeStr=Inherit: Same as input
  Kp2 : Gain  Gain=Mu  SaturateOnIntegerOverflow=on  SampleTime=Ts  OutDataTypeStr=Inherit: Same as input  ParamDataTypeStr=Inherit: Same as input
  Kp3 : Gain  Gain=C  SaturateOnIntegerOverflow=on  SampleTime=Ts  OutDataTypeStr=Inherit: Same as input  ParamDataTypeStr=Inherit: Same as input
  Kp4 : Gain  Gain=C  SaturateOnIntegerOverflow=on  SampleTime=Ts  OutDataTypeStr=Inherit: Same as input  ParamDataTypeStr=Inherit: Same as input
  Nr->wm : Gain  Gain=pi/30  SaturateOnIntegerOverflow=on  SampleTime=Ts  OutDataTypeStr=Inherit: Same as input  ParamDataTypeStr=Inherit: Same as input
  Saturation2 : Saturate  UpperLimit=UpperLimit  LowerLimit=LowerLimit  SampleTime=Ts
  Sum1 : Sum  InputSameDT=on  SaturateOnIntegerOverflow=on  SampleTime=Ts  OutDataTypeStr=Inherit: Same as first input
  Sum2 : Sum  Inputs=++++-  InputSameDT=on  SaturateOnIntegerOverflow=on  SampleTime=Ts  OutDataTypeStr=Inherit: Same as first input
  Trigonometric Function : Trigonometry  Operator=tanh
  Out : Outport  SampleTime=Ts  InitialOutput=0  VectorParamsAs1DForOutWhenUnconnected=off
  wires:
  Kp4/1 -> Sum1/1
  Saturation2/1 -> Out/1
  Error/1 -> Nr->wm/1
  Kp1/1 -> Sum2/1
  Sum1/1 -> Trigonometric Function/1, Kp1/1
  Kp2/1 -> Sum2/2
  Kp3/1 -> Sum2/3
  Nr->wm/1 -> Kp4/1, Abs/1, Derivative/1
  Derivative/1 -> Sum1/2, Kp3/1
  Sum2/1 -> Discrete-Time Integrator/1
  1/D/1 -> Saturation2/1
  Discrete-Time Integrator/1 -> 1/D/1
  Dot Product/1 -> Kp2/1
  Abs/1 -> Dot Product/2
  Trigonometric Function/1 -> Dot Product/1
  Constant1/1 -> Sum2/5, Sum2/4

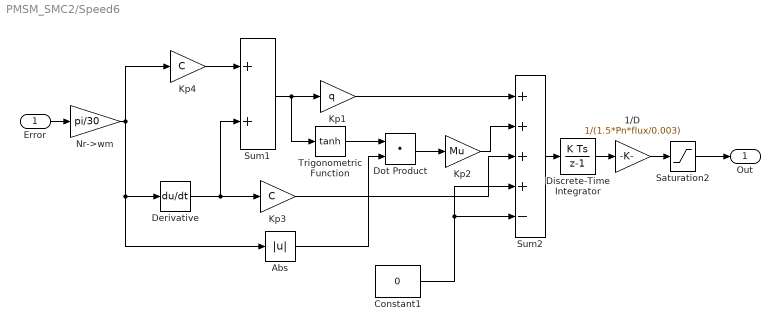
== system PMSM_SMC2/Speed6 ==
  Error : Inport  SampleTime=Ts
  1/D : Gain  Gain=1/(1.5*Pn*flux/0.003)  SaturateOnIntegerOverflow=on  SampleTime=Ts  OutDataTypeStr=Inherit: Same as input  ParamDataTypeStr=Inherit: Same as input
  Abs : Abs  SaturateOnIntegerOverflow=off
  Constant1 : Constant  Value=0
  Derivative : Derivative
  Discrete-Time Integrator : DiscreteIntegrator  InitialCondition=0.001  SampleTime=Ts  ICPrevOutput=DiscIntNeverNeededParam  ICPrevScaledInput=DiscIntNeverNeededParam
  Dot Product : DotProduct  OutDataTypeStr=Inherit: Inherit via internal rule
  Kp1 : Gain  Gain=q  SaturateOnIntegerOverflow=on  SampleTime=Ts  OutDataTypeStr=Inherit: Same as input  ParamDataTypeStr=Inherit: Same as input
  Kp2 : Gain  Gain=Mu  SaturateOnIntegerOverflow=on  SampleTime=Ts  OutDataTypeStr=Inherit: Same as input  ParamDataTypeStr=Inherit: Same as input
  Kp3 : Gain  Gain=C  SaturateOnIntegerOverflow=on  SampleTime=Ts  OutDataTypeStr=Inherit: Same as input  ParamDataTypeStr=Inherit: Same as input
  Kp4 : Gain  Gain=C  SaturateOnIntegerOverflow=on  SampleTime=Ts  OutDataTypeStr=Inherit: Same as input  ParamDataTypeStr=Inherit: Same as input
  Nr->wm : Gain  Gain=pi/30  SaturateOnIntegerOverflow=on  SampleTime=Ts  OutDataTypeStr=Inherit: Same as input  ParamDataTypeStr=Inherit: Same as input
  Saturation2 : Saturate  UpperLimit=UpperLimit  LowerLimit=LowerLimit  SampleTime=Ts
  Sum1 : Sum  InputSameDT=on  SaturateOnIntegerOverflow=on  SampleTime=Ts  OutDataTypeStr=Inherit: Same as first input
  Sum2 : Sum  Inputs=++++-  InputSameDT=on  SaturateOnIntegerOverflow=on  SampleTime=Ts  OutDataTypeStr=Inherit: Same as first input
  Trigonometric Function : Trigonometry  Operator=tanh
  Out : Outport  SampleTime=Ts  InitialOutput=0  VectorParamsAs1DForOutWhenUnconnected=off
  wires:
  Kp4/1 -> Sum1/1
  Saturation2/1 -> Out/1
  Error/1 -> Nr->wm/1
  Kp1/1 -> Sum2/1
  Sum1/1 -> Trigonometric Function/1, Kp1/1
  Kp2/1 -> Sum2/2
  Kp3/1 -> Sum2/3
  Nr->wm/1 -> Kp4/1, Abs/1, Derivative/1
  Derivative/1 -> Sum1/2, Kp3/1
  Sum2/1 -> Discrete-Time Integrator/1
  1/D/1 -> Saturation2/1
  Discrete-Time Integrator/1 -> 1/D/1
  Dot Product/1 -> Kp2/1
  Abs/1 -> Dot Product/2
  Trigonometric Function/1 -> Dot Product/1
  Constant1/1 -> Sum2/5, Sum2/4

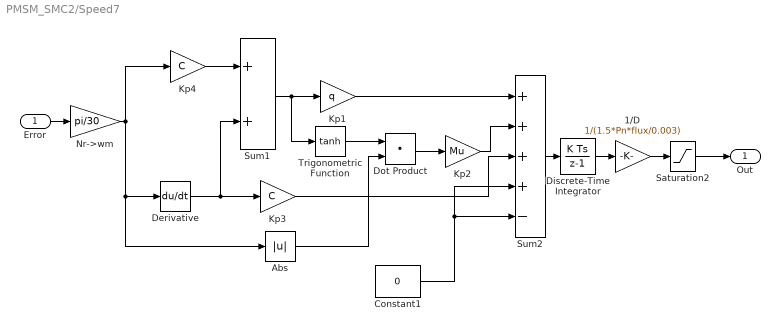
== system PMSM_SMC2/Speed7 ==
  Error : Inport  SampleTime=Ts
  1/D : Gain  Gain=1/(1.5*Pn*flux/0.003)  SaturateOnIntegerOverflow=on  SampleTime=Ts  OutDataTypeStr=Inherit: Same as input  ParamDataTypeStr=Inherit: Same as input
  Abs : Abs  SaturateOnIntegerOverflow=off
  Constant1 : Constant  Value=0
  Derivative : Derivative
  Discrete-Time Integrator : DiscreteIntegrator  InitialCondition=0.001  SampleTime=Ts  ICPrevOutput=DiscIntNeverNeededParam  ICPrevScaledInput=DiscIntNeverNeededParam
  Dot Product : DotProduct  OutDataTypeStr=Inherit: Inherit via internal rule
  Kp1 : Gain  Gain=q  SaturateOnIntegerOverflow=on  SampleTime=Ts  OutDataTypeStr=Inherit: Same as input  ParamDataTypeStr=Inherit: Same as input
  Kp2 : Gain  Gain=Mu  SaturateOnIntegerOverflow=on  SampleTime=Ts  OutDataTypeStr=Inherit: Same as input  ParamDataTypeStr=Inherit: Same as input
  Kp3 : Gain  Gain=C  SaturateOnIntegerOverflow=on  SampleTime=Ts  OutDataTypeStr=Inherit: Same as input  ParamDataTypeStr=Inherit: Same as input
  Kp4 : Gain  Gain=C  SaturateOnIntegerOverflow=on  SampleTime=Ts  OutDataTypeStr=Inherit: Same as input  ParamDataTypeStr=Inherit: Same as input
  Nr->wm : Gain  Gain=pi/30  SaturateOnIntegerOverflow=on  SampleTime=Ts  OutDataTypeStr=Inherit: Same as input  ParamDataTypeStr=Inherit: Same as input
  Saturation2 : Saturate  UpperLimit=UpperLimit  LowerLimit=LowerLimit  SampleTime=Ts
  Sum1 : Sum  InputSameDT=on  SaturateOnIntegerOverflow=on  SampleTime=Ts  OutDataTypeStr=Inherit: Same as first input
  Sum2 : Sum  Inputs=++++-  InputSameDT=on  SaturateOnIntegerOverflow=on  SampleTime=Ts  OutDataTypeStr=Inherit: Same as first input
  Trigonometric Function : Trigonometry  Operator=tanh
  Out : Outport  SampleTime=Ts  InitialOutput=0  VectorParamsAs1DForOutWhenUnconnected=off
  wires:
  Kp4/1 -> Sum1/1
  Saturation2/1 -> Out/1
  Error/1 -> Nr->wm/1
  Kp1/1 -> Sum2/1
  Sum1/1 -> Trigonometric Function/1, Kp1/1
  Kp2/1 -> Sum2/2
  Kp3/1 -> Sum2/3
  Nr->wm/1 -> Kp4/1, Abs/1, Derivative/1
  Derivative/1 -> Sum1/2, Kp3/1
  Sum2/1 -> Discrete-Time Integrator/1
  1/D/1 -> Saturation2/1
  Discrete-Time Integrator/1 -> 1/D/1
  Dot Product/1 -> Kp2/1
  Abs/1 -> Dot Product/2
  Trigonometric Function/1 -> Dot Product/1
  Constant1/1 -> Sum2/5, Sum2/4
